simulink subsystem "DiagnosticMode"  (R2023a)
settings: Solver=VariableStepAuto  StartTime=0.0  StopTime=10.0  RelTol=1e-3
settings Model: Creator=JesseJabezArendse  LastModifiedBy=Dylan Howard

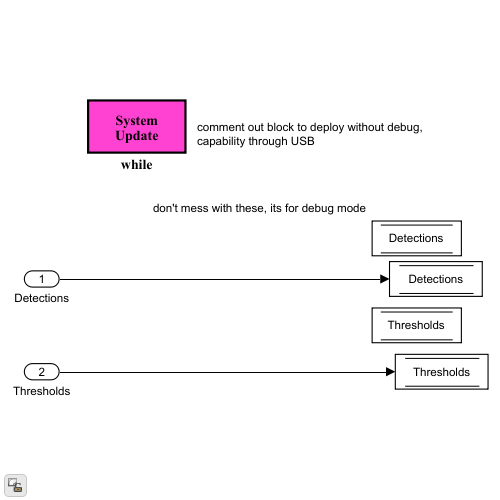
[thumbnail: Simulink's stored preview of the top-level diagram]
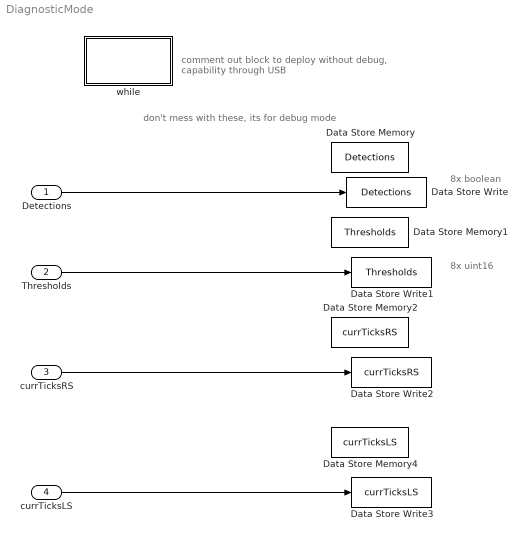
== system DiagnosticMode ==
  note: 8x uint16
  note: 8x boolean
  note: don't mess with these, its for debug mode
  note: comment out block to deploy without debug, capability through USB
  Detections : Inport
  Thresholds : Inport  Port=2
  currTicksRS : Inport  Port=3
  currTicksLS : Inport  Port=4
  Data Store Memory : DataStoreMemory  DataStoreName=Detections  WriteAfterWriteMsg=warning  ShowAdditionalParam=off  OutDataTypeStr=boolean  Dimensions=8
  Data Store Memory1 : DataStoreMemory  DataStoreName=Thresholds  WriteAfterWriteMsg=warning  ShowAdditionalParam=off  OutDataTypeStr=uint16  Dimensions=8
  Data Store Memory2 : DataStoreMemory  DataStoreName=currTicksRS  WriteAfterWriteMsg=warning  ShowAdditionalParam=off  OutDataTypeStr=int32  Dimensions=1
  Data Store Memory4 : DataStoreMemory  DataStoreName=currTicksLS  WriteAfterWriteMsg=warning  ShowAdditionalParam=off  OutDataTypeStr=int32  Dimensions=1
  Data Store Write : DataStoreWrite  DataStoreName=Detections  IndexOptions=Index vector (dialog)  Indices=1  OutputSizes=1
  Data Store Write1 : DataStoreWrite  DataStoreName=Thresholds  IndexOptions=Index vector (dialog)  Indices=1  OutputSizes=1
  Data Store Write2 : DataStoreWrite  DataStoreName=currTicksRS  IndexOptions=Index vector (dialog)  Indices=1  OutputSizes=1
  Data Store Write3 : DataStoreWrite  DataStoreName=currTicksLS  IndexOptions=Index vector (dialog)  Indices=1  OutputSizes=1
  while : Subsystem  Priority=0  TreatAsAtomicUnit=on  PartitionName=CustomWhilePartition  SystemSampleTime=0  mask(System Update){ShowInLibBrowser=0}
      mask prompts: ShowInLibBrowser "Simulink:masks:CustCodeMaskParam1_MP"
      settings: CopyFcn=cccopyfcn(gcb)  OpenFcn=ccopenfcn('System Update Function')  RTWFcnNameOpts=Use subsystem name  RTWFileNameOpts=Use function name
      mask Help: eval('feval(''rtwprivate'',''rtwhelpview'',''rtw_sys_update_block'')');
      mask DialogControl ShowInLibBrowser Prompt: Mask Parameter 1:
      mask Display: disp('System\nUpdate');
  wires:
  Thresholds/1 -> Data Store Write1/1
  Detections/1 -> Data Store Write/1
  currTicksRS/1 -> Data Store Write2/1
  currTicksLS/1 -> Data Store Write3/1

== system DiagnosticMode/while ==
